simulink model "buck_boost_converter_model"  (R2021a)
settings: Solver=VariableStepAuto  StartTime=0.0  StopTime=1  RelTol=1e-3
libraries: spsSeriesRLCBranchLib x6, spsDCVoltageSourceLib x2, spsDiodeLib x2, spsIGBTLib x2, spsSawtoothGeneratorLib x2, spsVoltageMeasurementLib x2, spspowerguiLib x1
settings Model: Creator=Pichau  LastModifiedBy=Pichau

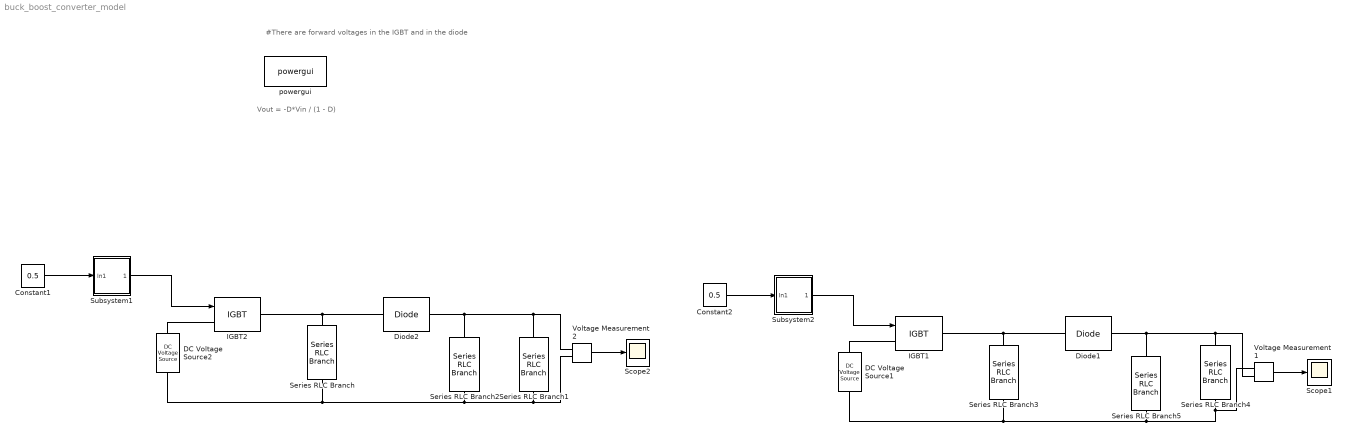
== system buck_boost_converter_model ==
  note: Vout = -D*Vin / (1 - D)
  note: #There are forward voltages in the IGBT and in the diode
  Constant1 : Constant  Value=0.5
  Constant2 : Constant  Value=0.5
  DC Voltage Source1 : spsDCVoltageSourceLib/DC Voltage Source  Amplitude=10  Measurements=None
  DC Voltage Source2 : spsDCVoltageSourceLib/DC Voltage Source  Amplitude=10  Measurements=None
  Diode1 : spsDiodeLib/Diode  Ron=0.001  Lon=0  Vf=0.8  IC=0  UseSnubber=0  Rs=500  Cs=250e-9  Measurements=off
  Diode2 : spsDiodeLib/Diode  Ron=0.001  Lon=0  Vf=0.8  IC=0  UseSnubber=0  Rs=500  Cs=250e-9  Measurements=off
  IGBT1 : spsIGBTLib/IGBT  Ron=0.001  Lon=0  Vf=1  Tf=1e-6  Tt=2e-6  IC=0  Rs=1e5  Cs=inf  Measurements=off
  IGBT2 : spsIGBTLib/IGBT  Ron=0.001  Lon=0  Vf=1  Tf=1e-6  Tt=2e-6  IC=0  Rs=1e5  Cs=inf  Measurements=off
  Scope1 : Scope
  Scope2 : Scope
  Series RLC Branch : spsSeriesRLCBranchLib/Series RLC Branch  LConnTagsString=__new0  RConnTagsString=__new0  BranchType=L  Resistance=1  Inductance=1e-3  SetiL0=off  InitialCurrent=0  Capacitance=1e-6  Setx0=off  InitialVoltage=0  Measurements=None
  Series RLC Branch1 : spsSeriesRLCBranchLib/Series RLC Branch  LConnTagsString=__new0  RConnTagsString=__new0  BranchType=R  Resistance=10  Inductance=1e-3  SetiL0=off  InitialCurrent=0  Capacitance=1e-6  Setx0=off  InitialVoltage=0  Measurements=None
  Series RLC Branch2 : spsSeriesRLCBranchLib/Series RLC Branch  LConnTagsString=__new0  RConnTagsString=__new0  BranchType=C  Resistance=10  Inductance=1e-3  SetiL0=off  InitialCurrent=0  Capacitance=10e-3  Setx0=off  InitialVoltage=0  Measurements=None
  Series RLC Branch3 : spsSeriesRLCBranchLib/Series RLC Branch  LConnTagsString=__new0  RConnTagsString=__new0  BranchType=L  Resistance=1  Inductance=1e-3  SetiL0=off  InitialCurrent=0  Capacitance=1e-6  Setx0=off  InitialVoltage=0  Measurements=None
  Series RLC Branch4 : spsSeriesRLCBranchLib/Series RLC Branch  LConnTagsString=__new0  RConnTagsString=__new0  BranchType=R  Resistance=10  Inductance=1e-3  SetiL0=off  InitialCurrent=0  Capacitance=1e-6  Setx0=off  InitialVoltage=0  Measurements=None
  Series RLC Branch5 : spsSeriesRLCBranchLib/Series RLC Branch  LConnTagsString=__new0  RConnTagsString=__new0  BranchType=C  Resistance=10  Inductance=1e-3  SetiL0=off  InitialCurrent=0  Capacitance=10e-3  Setx0=off  InitialVoltage=0  Measurements=None
  Subsystem1 : Subsystem
  Subsystem2 : Subsystem
  Voltage Measurement1 : spsVoltageMeasurementLib/Voltage Measurement  PhasorSimulation=off  OutputType=Complex  PSBequivalent=0
  Voltage Measurement2 : spsVoltageMeasurementLib/Voltage Measurement  PhasorSimulation=off  OutputType=Complex  PSBequivalent=0
  powergui : spspowerguiLib/powergui  Priority=1  SimulationMode=Discrete  SampleTime=5e-6  frequency=60  Iterations=50  frequencyindice=0  Pbase=100e6  ErrMax=1e-4  UnitsV=kV  UnitsW=MW  buscounter=0  FunctionMessages=off  echomessages=off  EnableUseOfTLC=off  CurrentSourceSwitches=off  DisableSnubberDevices=off  DisableRonSwitches=off  DisableVfSwitches=off  DisplayEquations=off  AutomaticDiscreteSolvers=off  SolverType=Tustin/Backward Euler (TBE)  Interpol=off  ExternalGateDelay=off  methode=off  Ts=100  x0status=blocks  SPID=on  SwTol=0  HookPort=off  NonlinearTolerance=1e-4  nMaxIteration=100  ContinueOnMaxIteration=off  RestoreLinks=warning  ResistiveCurrentMeasurement=off  Frange=[0:2:500]  Ylog=off  Xlog=on  ShowGrid=off  save=off  variable=ZData  structure=0  ZoomFFT=off  StartTime=0.0  cycles=1  DisplayStyle=1  fundamental=60  FreqAxis=off  MaxFrequency=1000  frequencyindicesteady=1  RmsSteady=1  display=off
  wires:
  Constant1/1 -> Subsystem1/1(In1)
  Subsystem1/1(Out1) -> IGBT2/1
  Voltage Measurement2/1 -> Scope2/1
  Subsystem2/1(Out1) -> IGBT1/1
  Constant2/1 -> Subsystem2/1(In1)
  Voltage Measurement1/1 -> Scope1/1
  connections:
  IGBT2/RConn1 -- Diode2/RConn1 -- Series RLC Branch/LConn1
  DC Voltage Source2/RConn1 -- IGBT2/LConn1
  Series RLC Branch/RConn1 -- Voltage Measurement2/LConn2 -- Series RLC Branch1/RConn1 -- Series RLC Branch2/RConn1 -- DC Voltage Source2/LConn1
  Series RLC Branch2/LConn1 -- Series RLC Branch1/LConn1 -- Voltage Measurement2/LConn1 -- Diode2/LConn1
  DC Voltage Source1/LConn1 -- Series RLC Branch3/RConn1 -- Voltage Measurement1/LConn1 -- Series RLC Branch4/LConn1 -- Series RLC Branch5/LConn1
  Series RLC Branch3/LConn1 -- IGBT1/RConn1 -- Diode1/RConn1
  Diode1/LConn1 -- Voltage Measurement1/LConn2 -- Series RLC Branch4/RConn1 -- Series RLC Branch5/RConn1
  DC Voltage Source1/RConn1 -- IGBT1/LConn1

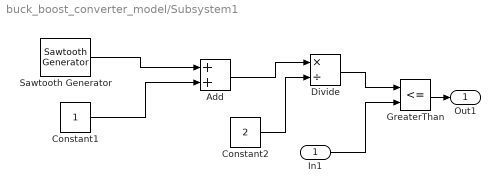
== system buck_boost_converter_model/Subsystem1 ==
  In1 : Inport
  Add : Sum
  Constant1 : Constant
  Constant2 : Constant  Value=2
  Divide : Product  Inputs=*/
  GreaterThan : RelationalOperator  Operator=<=  OutDataTypeStr=boolean  RndMeth=Simplest
  Sawtooth Generator : spsSawtoothGeneratorLib/Sawtooth Generator  Freq=5e3  Phase=0  Ts=0
  Out1 : Outport
  wires:
  Constant1/1 -> Add/2
  Add/1 -> Divide/1
  Sawtooth Generator/1 -> Add/1
  Constant2/1 -> Divide/2
  GreaterThan/1 -> Out1/1
  Divide/1 -> GreaterThan/1
  In1/1 -> GreaterThan/2

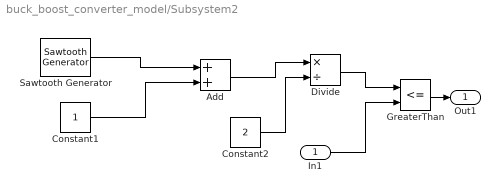
== system buck_boost_converter_model/Subsystem2 ==
  In1 : Inport
  Add : Sum
  Constant1 : Constant
  Constant2 : Constant  Value=2
  Divide : Product  Inputs=*/
  GreaterThan : RelationalOperator  Operator=<=  OutDataTypeStr=boolean  RndMeth=Simplest
  Sawtooth Generator : spsSawtoothGeneratorLib/Sawtooth Generator  Freq=5e3  Phase=0  Ts=0
  Out1 : Outport
  wires:
  Constant1/1 -> Add/2
  Add/1 -> Divide/1
  Sawtooth Generator/1 -> Add/1
  Constant2/1 -> Divide/2
  GreaterThan/1 -> Out1/1
  Divide/1 -> GreaterThan/1
  In1/1 -> GreaterThan/2
